simulink model "PID"  (R2025b)
settings: Solver=VariableStepAuto  StartTime=0.0  StopTime=10  RelTol=1e-3
settings Model: Creator=flipp  LastModifiedBy=flipp

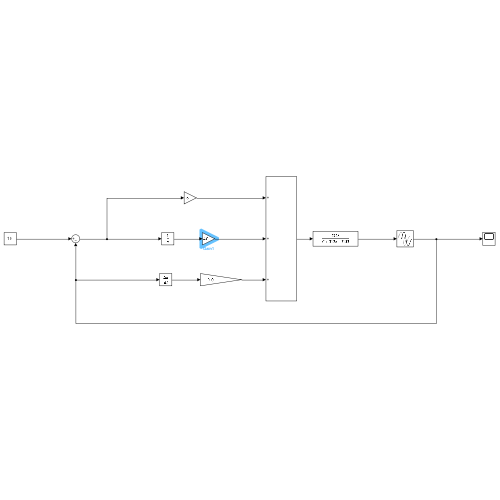
[thumbnail: Simulink's stored preview of the top-level diagram]
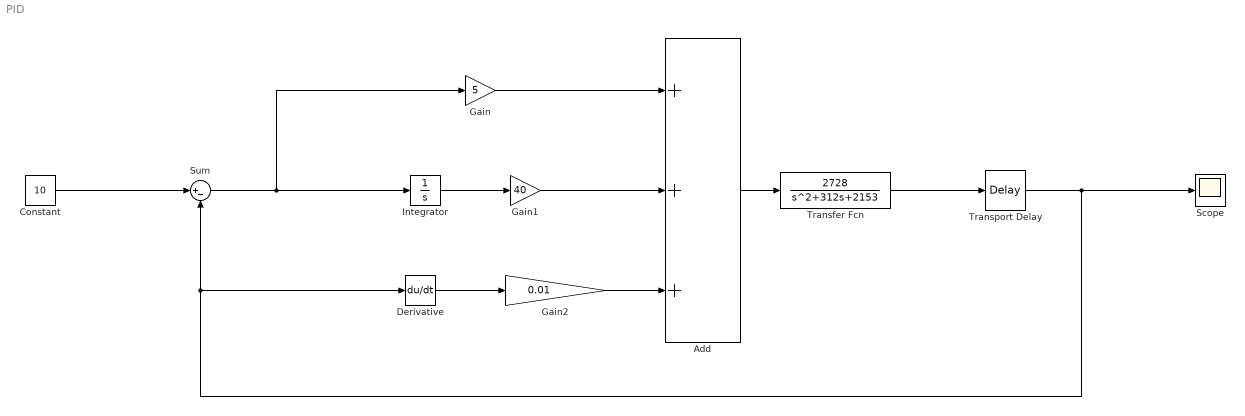
== system PID ==
  Add : Sum  Inputs=+++
  Constant : Constant  Value=10
  Derivative : Derivative
  Gain : Gain  Gain=5
  Gain1 : Gain  Gain=40
  Gain2 : Gain  Gain=0.01
  Integrator : Integrator  IgnoreLimit=on
  Scope : Scope
      settings: ActiveDisplayYMinimum=-17.860069908442519  ActiveDisplayYMaximum=6.8774102594875179
  Sum : Sum  Inputs=|+-
  Transfer Fcn : TransferFcn  Numerator=[2728]  Denominator=[1 312 2153]
  Transport Delay : TransportDelay
  wires:
  Constant/1 -> Sum/1
  Transfer Fcn/1 -> Transport Delay/1
  Transport Delay/1 -> Scope/1, Derivative/1, Sum/2
  Gain/1 -> Add/1
  Integrator/1 -> Gain1/1
  Derivative/1 -> Gain2/1
  Gain1/1 -> Add/2
  Gain2/1 -> Add/3
  Add/1 -> Transfer Fcn/1
  Sum/1 -> Gain/1, Integrator/1
